simulink model "P702_NI_SoftECU"  (R2019a)
settings: Solver=ode1  StartTime=0.0  StopTime=Inf  FixedStep=0.001  RelTol=1e-3  EnableMultiTasking=on
PreLoadFcn:
  | run '.\VeriStand_BlockSet\NIVeriStandAddPaths.m'
undefined symbols (not defined in the file or in its folder): magnitude
libraries: simulink x83, simulink_extras x1
(part 61 of 76)

== system P702_NI_SoftECU/SoftECU/ABS/Logic/Wheel Direction ==
  note: 0: forward
      | 1: backward
      | 2: unknown
      | 3: fault
  note: 0: forward
      | 1: backward
      | 2: unknown
      | 3: fault
  WhlRl_W_Meas : Inport
  WhlRr_W_Meas : Inport  Port=2
  Backward : Constant
  Backward1 : Constant
  Forward : Constant  Value=0
  Forward1 : Constant  Value=0
  If Action Subsystem1 : Subsystem  TreatAsAtomicUnit=on
  If Action Subsystem2 : Subsystem  TreatAsAtomicUnit=on
  If Action Subsystem3 : Subsystem  TreatAsAtomicUnit=on
  If Action Subsystem4 : Subsystem  TreatAsAtomicUnit=on
  If Action Subsystem5 : Subsystem  TreatAsAtomicUnit=on
  If Action Subsystem6 : Subsystem  TreatAsAtomicUnit=on
  If_Rl : If  IfExpression=u1 == 0  ElseIfExpressions=u1 > 0, u1<0  ShowElse=off
  If_Rr : If  IfExpression=u1 == 0  ElseIfExpressions=u1 > 0, u1<0  ShowElse=off
  Merge : Merge  Inputs=3  InitialOutput=[0]
  Merge1 : Merge  Inputs=3  InitialOutput=[0]
  Unknown : Constant  Value=2
  Unknown1 : Constant  Value=2
  WhlDirRl_D_Actl : Outport
  WhlDirRr_D_Actl : Outport  Port=2
  wires:
  If_Rl/1 -> If Action Subsystem1/Action
  If Action Subsystem3/1(Out1) -> Merge/3
  If Action Subsystem2/1(Out1) -> Merge/2
  If Action Subsystem1/1(Out1) -> Merge/1
  If_Rl/3 -> If Action Subsystem3/Action
  If_Rl/2 -> If Action Subsystem2/Action
  Backward/1 -> If Action Subsystem3/1(In1)
  Forward/1 -> If Action Subsystem2/1(In1)
  Unknown/1 -> If Action Subsystem1/1(In1)
  If_Rr/1 -> If Action Subsystem4/Action
  If Action Subsystem6/1(Out1) -> Merge1/3
  If Action Subsystem5/1(Out1) -> Merge1/2
  If Action Subsystem4/1(Out1) -> Merge1/1
  If_Rr/3 -> If Action Subsystem6/Action
  If_Rr/2 -> If Action Subsystem5/Action
  Backward1/1 -> If Action Subsystem6/1(In1)
  Forward1/1 -> If Action Subsystem5/1(In1)
  Unknown1/1 -> If Action Subsystem4/1(In1)
  Merge/1 -> WhlDirRl_D_Actl/1
  Merge1/1 -> WhlDirRr_D_Actl/1
  WhlRl_W_Meas/1 -> If_Rl/1
  WhlRr_W_Meas/1 -> If_Rr/1

== system P702_NI_SoftECU/SoftECU/ABS/Logic/WheelSpeedCounterFL ==
  Omega : Inport
  8BitCounter : Constant  Value=255
  Abs : Abs
  Compare To Constant : simulink/Logic and Bit Operations/Compare To Constant  relop=>=  const=100*2*3.14  OutDataTypeStr=boolean  ZeroCross=off
  Divide : Product  Inputs=*/
  Integrator : Integrator  ExternalReset=rising
  Math Function1 : Math  Operator=mod  SaturateOnIntegerOverflow=on
  Memory : Memory
  RadperTick : Constant  Value=0.05
  Saturation1 : Saturate  UpperLimit=327.65  LowerLimit=0  OutDataTypeStr=double
  Counter : Outport
  wires:
  Integrator/1 -> Memory/1, Divide/1
  Abs/1 -> Saturation1/1
  RadperTick/1 -> Divide/2
  Divide/1 -> Math Function1/1
  8BitCounter/1 -> Math Function1/2
  Saturation1/1 -> Integrator/1
  Omega/1 -> Abs/1
  Math Function1/1 -> Counter/1
  Compare To Constant/1 -> Integrator/2
  Memory/1 -> Compare To Constant/1

== system P702_NI_SoftECU/SoftECU/ABS/Logic/WheelSpeedCounterFR ==
  Omega : Inport
  8BitCounter : Constant  Value=255
  Abs : Abs
  Compare To Constant : simulink/Logic and Bit Operations/Compare To Constant  relop=>=  const=100*2*3.14  OutDataTypeStr=boolean  ZeroCross=off
  Divide : Product  Inputs=*/
  Integrator : Integrator  ExternalReset=rising
  Math Function1 : Math  Operator=mod  SaturateOnIntegerOverflow=on
  Memory : Memory
  RadperTick : Constant  Value=0.05
  Saturation1 : Saturate  UpperLimit=327.65  LowerLimit=0  OutDataTypeStr=double
  Counter : Outport
  wires:
  Memory/1 -> Compare To Constant/1
  Compare To Constant/1 -> Integrator/2
  Math Function1/1 -> Counter/1
  Omega/1 -> Abs/1
  Saturation1/1 -> Integrator/1
  8BitCounter/1 -> Math Function1/2
  Divide/1 -> Math Function1/1
  RadperTick/1 -> Divide/2
  Abs/1 -> Saturation1/1
  Integrator/1 -> Divide/1, Memory/1

== system P702_NI_SoftECU/SoftECU/ABS/Logic/WheelSpeedCounterRL ==
  Omega : Inport
  8BitCounter : Constant  Value=255
  Abs : Abs
  Compare To Constant : simulink/Logic and Bit Operations/Compare To Constant  relop=>=  const=100*2*3.14  OutDataTypeStr=boolean  ZeroCross=off
  Divide : Product  Inputs=*/
  Integrator : Integrator  ExternalReset=rising
  Math Function1 : Math  Operator=mod  SaturateOnIntegerOverflow=on
  Memory : Memory
  RadperTick : Constant  Value=0.05
  Saturation1 : Saturate  UpperLimit=327.65  LowerLimit=0  OutDataTypeStr=double
  Counter : Outport
  wires:
  Memory/1 -> Compare To Constant/1
  Compare To Constant/1 -> Integrator/2
  Math Function1/1 -> Counter/1
  Omega/1 -> Abs/1
  Saturation1/1 -> Integrator/1
  8BitCounter/1 -> Math Function1/2
  Divide/1 -> Math Function1/1
  RadperTick/1 -> Divide/2
  Abs/1 -> Saturation1/1
  Integrator/1 -> Divide/1, Memory/1

== system P702_NI_SoftECU/SoftECU/ABS/Logic/WheelSpeedCounterRR ==
  Omega : Inport
  8BitCounter : Constant  Value=255
  Abs : Abs
  Compare To Constant : simulink/Logic and Bit Operations/Compare To Constant  relop=>=  const=100*2*3.14  OutDataTypeStr=boolean  ZeroCross=off
  Divide : Product  Inputs=*/
  Integrator : Integrator  ExternalReset=rising
  Math Function1 : Math  Operator=mod  SaturateOnIntegerOverflow=on
  Memory : Memory
  RadperTick : Constant  Value=0.05
  Saturation1 : Saturate  UpperLimit=327.65  LowerLimit=0  OutDataTypeStr=double
  Counter : Outport
  wires:
  Integrator/1 -> Memory/1, Divide/1
  Abs/1 -> Saturation1/1
  RadperTick/1 -> Divide/2
  Divide/1 -> Math Function1/1
  8BitCounter/1 -> Math Function1/2
  Saturation1/1 -> Integrator/1
  Omega/1 -> Abs/1
  Math Function1/1 -> Counter/1
  Compare To Constant/1 -> Integrator/2
  Memory/1 -> Compare To Constant/1

== system P702_NI_SoftECU/SoftECU/ABS/Logic/veh_chksum1 ==
  vspd : Inport
  qf : Inport  Port=2
  ctr : Inport  Port=3
  Bitwise Operator : simulink/Logic and Bit Operations/Bitwise Operator  logicop=AND  UseBitMask=on  BitMask=bin2dec('1111111100000000')  BitMaskRealWorld=Stored Integer
  Bitwise Operator1 : simulink/Logic and Bit Operations/Bitwise Operator  logicop=AND  UseBitMask=on  BitMask=bin2dec('0000000011111111')  BitMaskRealWorld=Stored Integer
  Bitwise Operator2 : simulink/Logic and Bit Operations/Bitwise Operator  logicop=XOR  UseBitMask=off  NumInputPorts=2  BitMask=bin2dec('11011001')  BitMaskRealWorld=Stored Integer
  Bitwise Operator4 : simulink/Logic and Bit Operations/Bitwise Operator  logicop=AND  UseBitMask=on  BitMask=uint32(255)  BitMaskRealWorld=Stored Integer
  Bitwise Operator5 : simulink/Logic and Bit Operations/Bitwise Operator  logicop=AND  UseBitMask=on  BitMask=uint32(255)  BitMaskRealWorld=Stored Integer
  Data Type Conversion : DataTypeConversion  OutDataTypeStr=uint16
  Data Type Conversion1 : DataTypeConversion  OutDataTypeStr=uint16
  Data Type Conversion{2,4,7,9..10} (5 alike) : DataTypeConversion  OutDataTypeStr=uint8
  Hil_flag : Constant
  Shift Arithmetic : ArithShift  BitShiftNumber=8
  Sum : Sum  Inputs=++++
  Switch : Switch  Criteria=u2 > Threshold
  constant1 : Constant  Value=255
  chksum : Outport
  wires:
  Data Type Conversion2/1 -> Bitwise Operator2/2
  constant1/1 -> Data Type Conversion2/1
  Sum/1 -> Bitwise Operator2/1
  Data Type Conversion4/1 -> Sum/1
  Data Type Conversion10/1 -> Sum/4
  Data Type Conversion9/1 -> Sum/3
  Data Type Conversion7/1 -> Sum/2
  ctr/1 -> Data Type Conversion10/1
  qf/1 -> Data Type Conversion9/1
  Bitwise Operator5/1 -> Data Type Conversion7/1
  Bitwise Operator4/1 -> Data Type Conversion4/1
  Shift Arithmetic/1 -> Bitwise Operator4/1
  Bitwise Operator/1 -> Shift Arithmetic/1
  Bitwise Operator1/1 -> Bitwise Operator5/1
  Switch/1 -> Bitwise Operator/1, Bitwise Operator1/1
  vspd/1 -> Data Type Conversion/1, Data Type Conversion1/1
  Hil_flag/1 -> Switch/2
  Data Type Conversion1/1 -> Switch/3
  Data Type Conversion/1 -> Switch/1
  Bitwise Operator2/1 -> chksum/1

== system P702_NI_SoftECU/SoftECU/ABS/Logic/veh_chksum2 ==
  vspd : Inport
  qf : Inport  Port=2
  ctr : Inport  Port=3
  Bitwise Operator : simulink/Logic and Bit Operations/Bitwise Operator  logicop=AND  UseBitMask=on  BitMask=bin2dec('1111111100000000')  BitMaskRealWorld=Stored Integer
  Bitwise Operator1 : simulink/Logic and Bit Operations/Bitwise Operator  logicop=AND  UseBitMask=on  BitMask=bin2dec('0000000011111111')  BitMaskRealWorld=Stored Integer
  Bitwise Operator2 : simulink/Logic and Bit Operations/Bitwise Operator  logicop=XOR  UseBitMask=off  NumInputPorts=2  BitMask=bin2dec('11011001')  BitMaskRealWorld=Stored Integer
  Bitwise Operator4 : simulink/Logic and Bit Operations/Bitwise Operator  logicop=AND  UseBitMask=on  BitMask=uint32(255)  BitMaskRealWorld=Stored Integer
  Bitwise Operator5 : simulink/Logic and Bit Operations/Bitwise Operator  logicop=AND  UseBitMask=on  BitMask=uint32(255)  BitMaskRealWorld=Stored Integer
  Data Type Conversion : DataTypeConversion  OutDataTypeStr=uint16
  Data Type Conversion1 : DataTypeConversion  OutDataTypeStr=uint16
  Data Type Conversion{2,4,7,9..10} (5 alike) : DataTypeConversion  OutDataTypeStr=uint8
  Hil_flag : Constant
  Shift Arithmetic : ArithShift  BitShiftNumber=8
  Sum : Sum  Inputs=++++
  Switch : Switch  Criteria=u2 > Threshold
  constant1 : Constant  Value=255
  chksum : Outport
  wires:
  Bitwise Operator2/1 -> chksum/1
  Data Type Conversion/1 -> Switch/1
  Data Type Conversion1/1 -> Switch/3
  Hil_flag/1 -> Switch/2
  vspd/1 -> Data Type Conversion1/1, Data Type Conversion/1
  Switch/1 -> Bitwise Operator1/1, Bitwise Operator/1
  Bitwise Operator1/1 -> Bitwise Operator5/1
  Bitwise Operator/1 -> Shift Arithmetic/1
  Shift Arithmetic/1 -> Bitwise Operator4/1
  Bitwise Operator4/1 -> Data Type Conversion4/1
  Bitwise Operator5/1 -> Data Type Conversion7/1
  qf/1 -> Data Type Conversion9/1
  ctr/1 -> Data Type Conversion10/1
  Data Type Conversion7/1 -> Sum/2
  Data Type Conversion9/1 -> Sum/3
  Data Type Conversion10/1 -> Sum/4
  Data Type Conversion4/1 -> Sum/1
  Sum/1 -> Bitwise Operator2/1
  constant1/1 -> Data Type Conversion2/1
  Data Type Conversion2/1 -> Bitwise Operator2/2

== system P702_NI_SoftECU/SoftECU/ABS/Mapping/ABS_BrkBst_Data ==
  In1 : Inport
  Bus Creator7 : BusCreator  Inputs=3
  Bus Selector3 : BusSelector  OutputSignals=BrkTot_Tq_RqDrv,BrkTotTqRqDrv_No_Cs,BrkTotTqRqDrv_No_Cnt
  Gain : Gain
  Gain1 : Gain
  Gain2 : Gain
  Out1 : Outport
  wires:
  Bus Selector3/2 -> Gain1/1  "<BrkTotTqRqDrv_No_Cs>"
  Bus Selector3/1 -> Gain/1  "<BrkTot_Tq_RqDrv>"
  In1/1 -> Bus Selector3/1
  Bus Creator7/1 -> Out1/1  "ABS_BrkBst_Data"
  Gain1/1 -> Bus Creator7/2  "BrkTotTqRqDrv_No_Cs"
  Gain/1 -> Bus Creator7/1  "BrkTot_Tq_RqDrv"
  Bus Selector3/3 -> Gain2/1  "<BrkTotTqRqDrv_No_Cnt>"
  Gain2/1 -> Bus Creator7/3  "BrkTotTqRqDrv_No_Cnt"

== system P702_NI_SoftECU/SoftECU/ABS/Mapping/Accel_Data ==
  In1 : Inport
  Bus Creator10 : BusCreator  Inputs=2
  Bus Selector3 : BusSelector  OutputSignals=VehLong2_A_Actl,VehLat2_A_Actl
  Gain : Gain
  Gain1 : Gain
  Out1 : Outport
  wires:
  Gain/1 -> Bus Creator10/1  "VehLong2_A_Actl"
  Gain1/1 -> Bus Creator10/2  "VehLat2_A_Actl"
  Bus Creator10/1 -> Out1/1  "Accel_Data"
  In1/1 -> Bus Selector3/1
  Bus Selector3/1 -> Gain/1  "<VehLong2_A_Actl>"
  Bus Selector3/2 -> Gain1/1  "<VehLat2_A_Actl>"

== system P702_NI_SoftECU/SoftECU/ABS/Mapping/BrakeSnData_3 ==
  In1 : Inport
  Bus Creator12 : BusCreator  Inputs=4
  Bus Selector3 : BusSelector  OutputSignals=VehYawComp_W_Actl,VehOverGnd_V_Est,VehLongComp_A_Actl,VehLatComp_A_Actl
  Gain{,1..3} (4 alike) : Gain
  Out1 : Outport
  wires:
  Gain1/1 -> Bus Creator12/2  "VehOverGnd_V_Est"
  Gain/1 -> Bus Creator12/1  "VehYawComp_W_Actl"
  Gain2/1 -> Bus Creator12/3  "VehLongComp_A_Actl"
  Gain3/1 -> Bus Creator12/4  "VehLatComp_A_Actl"
  Bus Creator12/1 -> Out1/1  "BrakeSnData_3"
  In1/1 -> Bus Selector3/1
  Bus Selector3/3 -> Gain2/1  "<VehLongComp_A_Actl>"
  Bus Selector3/2 -> Gain1/1  "<VehOverGnd_V_Est>"
  Bus Selector3/4 -> Gain3/1  "<VehLatComp_A_Actl>"
  Bus Selector3/1 -> Gain/1  "<VehYawComp_W_Actl>"

== system P702_NI_SoftECU/SoftECU/ABS/Mapping/BrakeSnData_4 ==
  In1 : Inport
  Bus Creator : BusCreator  Inputs=3
  Bus Selector3 : BusSelector  OutputSignals=VehVertComp_A_Actl,VehRolComp_W_Actl,BrkTot_Tq_RqDrv
  Gain : Gain
  Gain1 : Gain
  Gain2 : Gain
  Out1 : Outport
  wires:
  Gain/1 -> Bus Creator/1  "VehVertComp_A_Actl"
  Bus Creator/1 -> Out1/1  "BrakeSnData_4"
  Gain1/1 -> Bus Creator/2  "VehRolComp_W_Actl"
  Bus Selector3/1 -> Gain/1  "<VehVertComp_A_Actl>"
  Bus Selector3/2 -> Gain1/1  "<VehRolComp_W_Actl>"
  In1/1 -> Bus Selector3/1
  Bus Selector3/3 -> Gain2/1  "<BrkTot_Tq_RqDrv>"
  Gain2/1 -> Bus Creator/3  "BrkTot_Tq_Actl"

== system P702_NI_SoftECU/SoftECU/ABS/Mapping/BrakeSnData_5 ==
  In1 : Inport
  Bus Creator : BusCreator  Inputs=1
  Bus Selector3 : BusSelector  OutputSignals=SteWhlComp_An_Est
  Gain : Gain
  Out1 : Outport
  wires:
  In1/1 -> Bus Selector3/1
  Bus Selector3/1 -> Gain/1  "<SteWhlComp_An_Est>"
  Bus Creator/1 -> Out1/1  "BrakeSnData_5"
  Gain/1 -> Bus Creator/1  "SteWhlComp_An_Est"

== system P702_NI_SoftECU/SoftECU/ABS/Mapping/BrakeSysFeatures ==
  In1 : Inport
  Bus Creator5 : BusCreator  Inputs=3
  Bus Selector3 : BusSelector  OutputSignals=Veh_V_ActlBrk,VehVActlBrk_No_Cs,VehVActlBrk_No_Cnt
  Gain : Gain
  Gain1 : Gain
  Gain2 : Gain
  Out1 : Outport
  wires:
  Bus Creator5/1 -> Out1/1  "BrakeSysFeatures"
  Gain/1 -> Bus Creator5/1  "Veh_V_ActlBrk"
  In1/1 -> Bus Selector3/1
  Bus Selector3/1 -> Gain/1  "<Veh_V_ActlBrk>"
  Bus Selector3/2 -> Gain1/1  "<VehVActlBrk_No_Cs>"
  Bus Selector3/3 -> Gain2/1  "<VehVActlBrk_No_Cnt>"
  Gain1/1 -> Bus Creator5/2  "VehVActlBrk_No_Cs"
  Gain2/1 -> Bus Creator5/3  "VehVActlBrk_No_Cnt"

== system P702_NI_SoftECU/SoftECU/ABS/Mapping/BrakeSysFeatures_2 ==
  In1 : Inport
  Bus Creator7 : BusCreator  Inputs=3
  Bus Selector3 : BusSelector  OutputSignals=BpedMove_D_Actl,BpedMove_No_Cs,BpedMove_No_Cnt
  Gain : Gain
  Gain1 : Gain
  Gain2 : Gain
  Out1 : Outport
  wires:
  Gain2/1 -> Bus Creator7/3  "BpedMove_No_Cnt"
  Bus Selector3/3 -> Gain2/1  "<BpedMove_No_Cnt>"
  Gain/1 -> Bus Creator7/1  "BpedMove_D_Actl"
  Gain1/1 -> Bus Creator7/2  "BpedMove_No_Cs"
  Bus Creator7/1 -> Out1/1  "BrakeSysFeatures_2"
  In1/1 -> Bus Selector3/1
  Bus Selector3/1 -> Gain/1  "<BpedMove_D_Actl>"
  Bus Selector3/2 -> Gain1/1  "<BpedMove_No_Cs>"

== system P702_NI_SoftECU/SoftECU/ABS/Mapping/DesiredTorqBrk ==
  In1 : Inport
  Bus Creator11 : BusCreator  Inputs=10
  Bus Selector3 : BusSelector  OutputSignals=AccBrkPrchgActv_B_Actl,AccBrkActv_B_Actl,AccStopActv_B_ActlBrk,CmbbBrkPrchg_B_Actl,CmbbBaSensInc_B_Actl,CmbbBrkDecel_B_Actl,VehicleStationary,VehLongOvrGnd_A_Est,AccBrkTotTqMn_B_Actl
  Gain{,1..9} (10 alike) : Gain
  Out1 : Outport
  wires:
  Gain8/1 -> Bus Creator11/9  "VehLongOvrGnd_A_Est"
  Bus Creator11/1 -> Out1/1  "DesiredTorqBrk"
  Gain1/1 -> Bus Creator11/2  "AccBrkActv_B_Actl"
  Gain/1 -> Bus Creator11/1  "AccBrkPrchgActv_B_Actl"
  Gain2/1 -> Bus Creator11/3  "AccStopActv_B_ActlBrk"
  Gain3/1 -> Bus Creator11/4  "CmbbBrkPrchg_B_Actl"
  Gain4/1 -> Bus Creator11/5  "CmbbBaSensInc_B_Actl"
  Gain5/1 -> Bus Creator11/6  "CmbbBrkDecel_B_Actl"
  Gain6/1 -> Bus Creator11/7  "VehicleStationary"
  In1/1 -> Bus Selector3/1
  Bus Selector3/4 -> Gain3/1  "<CmbbBrkPrchg_B_Actl>"
  Bus Selector3/2 -> Gain1/1  "<AccBrkActv_B_Actl>"
  Bus Selector3/1 -> Gain/1  "<AccBrkPrchgActv_B_Actl>"
  Bus Selector3/3 -> Gain2/1  "<AccStopActv_B_ActlBrk>"
  Bus Selector3/5 -> Gain4/1  "<CmbbBaSensInc_B_Actl>"
  Bus Selector3/6 -> Gain5/1  "<CmbbBrkDecel_B_Actl>"
  Bus Selector3/7 -> Gain7/1, Gain6/1  "<VehicleStationary>"
  Bus Selector3/8 -> Gain8/1  "<VehLongOvrGnd_A_Est>"
  Bus Selector3/9 -> Gain9/1  "<AccBrkTotTqMn_B_Actl>"
  Gain9/1 -> Bus Creator11/10  "AccBrkTotTqMn_B_Actl"
  Gain7/1 -> Bus Creator11/8  "VehStop_D_Stat"

== system P702_NI_SoftECU/SoftECU/ABS/Mapping/ToCarSim ==
  In1 : Inport
  Bus Creator : BusCreator  Inputs=1
  Bus Selector3 : BusSelector  OutputSignals=ABSPhysical.MCPressure
  Out1 : Outport
  wires:
  In1/1 -> Bus Selector3/1
  Bus Creator/1 -> Out1/1  "ToCarSim"
  Bus Selector3/1 -> Bus Creator/1  "<MCPressure>"

== system P702_NI_SoftECU/SoftECU/ABS/Mapping/WheelData ==
  In1 : Inport
  Bus Creator7 : BusCreator  Inputs=2
  Bus Selector3 : BusSelector  OutputSignals=WhlDirRl_D_Actl,WhlDirRr_D_Actl
  Gain : Gain
  Gain1 : Gain
  Out1 : Outport
  wires:
  Gain/1 -> Bus Creator7/1  "WhlDirRl_D_Actl"
  Gain1/1 -> Bus Creator7/2  "WhlDirRr_D_Actl"
  Bus Creator7/1 -> Out1/1  "WheelData"
  In1/1 -> Bus Selector3/1
  Bus Selector3/1 -> Gain/1  "<WhlDirRl_D_Actl>"
  Bus Selector3/2 -> Gain1/1  "<WhlDirRr_D_Actl>"

== system P702_NI_SoftECU/SoftECU/ABS/Mapping/WheelSpeed ==
  In1 : Inport
  Bus Creator6 : BusCreator  Inputs=8
  Bus Selector3 : BusSelector  OutputSignals=WhlFl_W_Meas,WhlFr_W_Meas,WhlRl_W_Meas,WhlRr_W_Meas,WhlRotatFl_No_Cnt,WhlRotatFr_No_Cnt,WhlRotatRl_No_Cnt,WhlRotatRr_No_Cnt
  Gain{,1..7} (8 alike) : Gain
  Out1 : Outport
  wires:
  In1/1 -> Bus Selector3/1
  Gain/1 -> Bus Creator6/1  "WhlFl_W_Meas"
  Gain1/1 -> Bus Creator6/2  "WhlFr_W_Meas"
  Gain2/1 -> Bus Creator6/3  "WhlRl_W_Meas"
  Gain3/1 -> Bus Creator6/4  "WhlRr_W_Meas"
  Bus Creator6/1 -> Out1/1  "WheelSpeed"
  Bus Selector3/2 -> Gain1/1  "<WhlFr_W_Meas>"
  Bus Selector3/1 -> Gain/1  "<WhlFl_W_Meas>"
  Bus Selector3/3 -> Gain2/1  "<WhlRl_W_Meas>"
  Bus Selector3/4 -> Gain3/1  "<WhlRr_W_Meas>"
  Bus Selector3/8 -> Gain7/1  "<WhlRotatRr_No_Cnt>"
  Bus Selector3/7 -> Gain6/1  "<WhlRotatRl_No_Cnt>"
  Bus Selector3/5 -> Gain4/1  "<WhlRotatFl_No_Cnt>"
  Bus Selector3/6 -> Gain5/1  "<WhlRotatFr_No_Cnt>"
  Gain7/1 -> Bus Creator6/8  "WhlRotatRr_No_Cnt"
  Gain6/1 -> Bus Creator6/7  "WhlRotatRl_No_Cnt"
  Gain4/1 -> Bus Creator6/5  "WhlRotatFl_No_Cnt"
  Gain5/1 -> Bus Creator6/6  "WhlRotatFr_No_Cnt"

== system P702_NI_SoftECU/SoftECU/ABS/Mapping/Yaw_Data ==
  In1 : Inport
  Bus Creator9 : BusCreator  Inputs=1
  Bus Selector3 : BusSelector  OutputSignals=VehYaw_W_Actl
  Gain : Gain
  Out1 : Outport
  wires:
  Gain/1 -> Bus Creator9/1  "VehYaw_W_Actl"
  Bus Creator9/1 -> Out1/1  "Yaw_Data"
  In1/1 -> Bus Selector3/1
  Bus Selector3/1 -> Gain/1  "<VehYaw_W_Actl>"

== system P702_NI_SoftECU/SoftECU/BCM/Logic/GGCC_Config_Mgmt_ID ==
  note: VIN:
      | 17 characters as ASCII vector
      |
      | AxleRatio:
      | Min = 0.01
      | Max = 655.34
      | Res = 0.01
      |
      | TireCircumference:
      | Min = 1
      | Max = 65534
      | Res = 1
      | Unit = mm
      |
      | RCMAuxId:
      | 2 bytes
      |
      | LowSpeedCmbbCfg:
      | 1 = Without Low Speed CMbB
      | 2 = Low Speed CMbB
      |
      | FuelCfg:
      | 1 = Gasoline
      | 2 = Diesel
      | 3 = Gas/Electric Hybrid
      | 4 = Hydrogen Fuel Cell
      | 5 = Diesel/Electric Hybrid
      | 6 = Compressed Natural Gas
      | 7 = Electric Only
      |
      | AccCfg:
      | 1 = Without Cruise Control
      | 2 = Cruise Control
      | 3 = Adaptive Cruise Control
      | 4 = Adaptive Cruise Control Stop & Go
      |
      | DriveCfg:
      | 1 = Without 4WD
      | 2 = Selectable 4WD
      | 3 = Permanent 4WD
      | 4 = AWD
      |
      | DriveSideCfg:
      | 1 = Left Hand Drive
      | 2 = Right Hand Drive
      |
      | GearboxCfg:
      | 1 = Manual
      | 2 = Automatic
  note: KunalP: VINCalculation Modified by BrianTamm
  AccCfg : Constant  Value=4
  AxleRatio : Constant  Value=3.21
  Bus Creator : BusCreator  Inputs=8
  Bus Creator1 : BusCreator  Inputs=1
  CmbbCfg : Constant  Value=3
  DriveCfg : Constant
  DriveSideCfg : Constant
  FuelCfg : Constant
  GearboxCfg : Constant  Value=2
  LowSpeedCmbbCfg : Constant
  MUX_delay : UnitDelay  SampleTime=0.2  HasFrameUpgradeWarning=on
  RCMAuxId : Constant  Value=hex2dec('20C3')
  Rate Transition1 : RateTransition
  Terminator{,1..5} (6 alike) : Terminator
  TireCircumference : Constant  Value=2534
  VIN : Constant  Value=double('ABCDEFGHIJKLMNOPQ')  VectorParams1D=off  OutDataTypeStr=double
  VIN_Calculation : MATLAB Function  TreatAsAtomicUnit=on
  Out1 : Outport
  wires:
  Bus Creator1/1 -> Out1/1  "GGCC_Config_Mgmt_ID"
  MUX_delay/1 -> VIN_Calculation/12(MUX_in)
  VIN_Calculation/9(MUX_out) -> Rate Transition1/1
  VIN_Calculation/2(Byte_1) -> Bus Creator/2
  VIN_Calculation/3(Byte_2) -> Bus Creator/3
  VIN_Calculation/4(Byte_3) -> Bus Creator/4
  VIN_Calculation/5(Byte_4) -> Bus Creator/5
  VIN_Calculation/6(Byte_5) -> Bus Creator/6
  VIN_Calculation/7(Byte_6) -> Bus Creator/7
  VIN_Calculation/8(Byte_7) -> Bus Creator/8
  Rate Transition1/1 -> MUX_delay/1
  Bus Creator/1 -> Bus Creator1/1  "VehicleGGCCData"
  VIN_Calculation/1(Byte_0) -> Bus Creator/1
  VIN/1 -> VIN_Calculation/1(VIN)
  AxleRatio/1 -> VIN_Calculation/2(AxleRatio)
  TireCircumference/1 -> VIN_Calculation/3(TireCircumference)
  RCMAuxId/1 -> VIN_Calculation/4(RCMAuxId)
  LowSpeedCmbbCfg/1 -> VIN_Calculation/5(LowSpeedCmbbCfg)
  FuelCfg/1 -> VIN_Calculation/6(FuelCfg)
  AccCfg/1 -> VIN_Calculation/7(AccCfg)
  CmbbCfg/1 -> VIN_Calculation/8(CmbbCfg)
  DriveCfg/1 -> VIN_Calculation/9(DriveCfg)
  DriveSideCfg/1 -> VIN_Calculation/10(DriveSideCfg)
  GearboxCfg/1 -> VIN_Calculation/11(GearboxCfg)
  VIN_Calculation/10(C000_out) -> Terminator/1
  VIN_Calculation/11(C100_out) -> Terminator1/1
  VIN_Calculation/12(C101_out) -> Terminator2/1
  VIN_Calculation/13(C102_out) -> Terminator3/1
  VIN_Calculation/14(C104_out) -> Terminator4/1
  VIN_Calculation/15(C110_out) -> Terminator5/1

== system P702_NI_SoftECU/SoftECU/BCM/Logic/IgnitionState ==
  In : Inport
  Accessory : Constant  Value=2
  Bus Creator : BusCreator  Inputs=1
  Constant : Constant  Value=2
  If : If  IfExpression=u1 <= 0  ElseIfExpressions=u1 == 1, u1 == 2, u1 == 3
  If Action Subsystem1 : Subsystem  TreatAsAtomicUnit=on
  If Action Subsystem2 : Subsystem  TreatAsAtomicUnit=on
  If Action Subsystem3 : Subsystem  TreatAsAtomicUnit=on
  If Action Subsystem4 : Subsystem  TreatAsAtomicUnit=on
  If Action Subsystem5 : Subsystem  TreatAsAtomicUnit=on
  Invalid : Constant  Value=15
  Merge : Merge  Inputs=5  InitialOutput=[0]
  Off : Constant
  Run : Constant  Value=4
  Start : Constant  Value=8
  Terminator : Terminator
  Out : Outport
  wires:
  Merge/1 -> Bus Creator/1  "IgnitionStatus"
  Off/1 -> If Action Subsystem1/1(In1)
  Accessory/1 -> If Action Subsystem2/1(In1)
  Run/1 -> If Action Subsystem3/1(In1)
  Start/1 -> If Action Subsystem4/1(In1)
  Invalid/1 -> If Action Subsystem5/1(In1)
  If/2 -> If Action Subsystem2/Action
  If/5 -> If Action Subsystem5/Action
  If/3 -> If Action Subsystem3/Action
  If/4 -> If Action Subsystem4/Action
  If Action Subsystem1/1(Out1) -> Merge/1
  If Action Subsystem2/1(Out1) -> Merge/2
  If Action Subsystem3/1(Out1) -> Merge/3
  If Action Subsystem4/1(Out1) -> Merge/4
  If Action Subsystem5/1(Out1) -> Merge/5
  If/1 -> If Action Subsystem1/Action
  In/1 -> Terminator/1
  Constant/1 -> If/1
  Bus Creator/1 -> Out/1  "Ignition"

== system P702_NI_SoftECU/SoftECU/BCM/Logic/OdometerValues ==
  In : Inport
  Bus Creator : BusCreator  Inputs=2
  Bus Selector2 : BusSelector  OutputSignals=s_Vehicle[m]
  Constant : Constant  Value=1000
  Constant2 : Constant  Value=1000
  Derivative : Derivative
  Divide : Product  Inputs=*/
  If : If  IfExpression=u1 <= 0
  If Action Subsystem1 : Subsystem  TreatAsAtomicUnit=on
  If Action Subsystem4 : Subsystem  TreatAsAtomicUnit=on
  Merge : Merge  InitialOutput=[0]
  Off : Constant  Value=0
  Start : Constant
  Start1 : Constant  Value=0.5
  Sum : Sum  Inputs=++|
  Variable Time Delay : VariableTransportDelay  MaximumDelay=10  MaximumPoints=10240
  Out : Outport
  wires:
  In/1 -> Bus Selector2/1
  Bus Creator/1 -> Out/1  "OdometerValues"
  Bus Selector2/1 -> Divide/1  "<s_Vehicle[m]>"
  Constant/1 -> Divide/2
  Divide/1 -> Sum/2
  Sum/1 -> Bus Creator/1, Derivative/1  "OdometerMasterValue"
  Merge/1 -> Variable Time Delay/1
  Off/1 -> If Action Subsystem1/1(In1)
  Start/1 -> If Action Subsystem4/1(In1)
  If/2 -> If Action Subsystem4/Action
  If Action Subsystem1/1(Out1) -> Merge/1
  If Action Subsystem4/1(Out1) -> Merge/2
  If/1 -> If Action Subsystem1/Action
  Derivative/1 -> If/1
  Start1/1 -> Variable Time Delay/2
  Variable Time Delay/1 -> Bus Creator/2  "OdometerMasterValue_UB"
  Constant2/1 -> Sum/1

== system P702_NI_SoftECU/SoftECU/BCM/Mapping/BodyEngGateway_2 ==
  In1 : Inport
  Ground : Ground
  Terminator : Terminator
  Out1 : Outport
  wires:
  In1/1 -> Terminator/1
  Ground/1 -> Out1/1

== system P702_NI_SoftECU/SoftECU/BCM/Mapping/BodyInfo_3 ==
  In : Inport
  Bus Creator : BusCreator  Inputs=1
  Bus Selector : BusSelector  OutputSignals=Ignition.IgnitionStatus
  Gain : Gain
  Out : Outport
  wires:
  Gain/1 -> Bus Creator/1  "Ignition_Status"
  Bus Creator/1 -> Out/1  "BodyInfo_3"
  In/1 -> Bus Selector/1
  Bus Selector/1 -> Gain/1  "<IgnitionStatus>"

== system P702_NI_SoftECU/SoftECU/BCM/Mapping/Cluster_Info1 ==
  In : Inport
  Bus Creator : BusCreator  Inputs=2
  Bus Selector2 : BusSelector  OutputSignals=OdometerValues.OdometerMasterValue,OdometerValues.OdometerMasterValue_UB
  Gain : Gain
  Gain1 : Gain
  Out : Outport
  wires:
  Gain1/1 -> Bus Creator/2  "OdometerMasterValue_UB"
  Gain/1 -> Bus Creator/1  "OdometerMasterValue"
  Bus Selector2/2 -> Gain1/1  "<OdometerMasterValue_UB>"
  Bus Selector2/1 -> Gain/1  "<OdometerMasterValue>"
  Bus Creator/1 -> Out/1  "Cluster_Info1"
  In/1 -> Bus Selector2/1

== system P702_NI_SoftECU/SoftECU/BCM/Mapping/GGCC_Config_Mgmt_ID ==
  In1 : Inport
  Bus Creator : BusCreator  Inputs=8
  Bus Selector : BusSelector  OutputSignals=GGCC_Config_Mgmt_ID.VehicleGGCCData.Byte_0,GGCC_Config_Mgmt_ID.VehicleGGCCData.Byte_1,GGCC_Config_Mgmt_ID.VehicleGGCCData.Byte_2,GGCC_Config_Mgmt_ID.VehicleGGCCData.Byte_3,GGCC_Config_Mgmt_ID.VehicleGGCCData.Byte_4,GGCC_Config_Mgmt_ID.VehicleGGCCData.Byte_5,GGCC_Config_Mgmt_ID.VehicleGGCCData.Byte_6,GGCC_Config_Mgmt_ID.VehicleGGCCData.Byte_7
  Out1 : Outport
  wires:
  In1/1 -> Bus Selector/1
  Bus Creator/1 -> Out1/1  "GGCC_Config_Mgmt_ID"
  Bus Selector/3 -> Bus Creator/3  "<Byte_2>"
  Bus Selector/6 -> Bus Creator/6  "<Byte_5>"
  Bus Selector/4 -> Bus Creator/4  "<Byte_3>"
  Bus Selector/2 -> Bus Creator/2  "<Byte_1>"
  Bus Selector/8 -> Bus Creator/8  "<Byte_7>"
  Bus Selector/7 -> Bus Creator/7  "<Byte_6>"
  Bus Selector/5 -> Bus Creator/5  "<Byte_4>"
  Bus Selector/1 -> Bus Creator/1  "<Byte_0>"

== system P702_NI_SoftECU/SoftECU/BCM/Mapping/Gear_Shift_By_Wire ==
  In1 : Inport
  Ground : Ground
  Terminator : Terminator
  Out1 : Outport
  wires:
  In1/1 -> Terminator/1
  Ground/1 -> Out1/1

== system P702_NI_SoftECU/SoftECU/BCM/Mapping/KeyStates ==
  In : Inport
  Ground : Ground
  Terminator : Terminator
  Out : Outport
  wires:
  In/1 -> Terminator/1
  Ground/1 -> Out/1

== system P702_NI_SoftECU/SoftECU/BCM/Mapping/Personality_BCM2_Data ==
  note: Han: the update rate of Personality_BCM2_Data is 1 Hz
  Bus Creator : BusCreator  Inputs=1
  Counter Limited : simulink/Sources/Counter Limited  uplimit=255  tsamp=1
  Data Type Conversion : DataTypeConversion  OutDataTypeStr=uint8
  Out : Outport
  wires:
  Bus Creator/1 -> Out/1  "Personality_BCM2_Data"
  Counter Limited/1 -> Data Type Conversion/1
  Data Type Conversion/1 -> Bus Creator/1  "RecallEvent_No_Cnt"

== system P702_NI_SoftECU/SoftECU/DSMC/Logic/Compute_DrvEngageLevel_No_Cs ==
  DrvEngLvlConfid_D_Stat : Inport
  DrvEngageLevel_D_Stat : Inport  Port=2
  DrvEngageLevel_No_Cnt : Inport  Port=3
  Bitwise Operator1 : simulink/Logic and Bit Operations/Bitwise Operator  logicop=AND  UseBitMask=on  BitMask=bin2dec('0000000011111111')  BitMaskRealWorld=Stored Integer
  Bitwise Operator2 : simulink/Logic and Bit Operations/Bitwise Operator  logicop=NOT  UseBitMask=off  BitMask=bin2dec('11011001')  BitMaskRealWorld=Stored Integer
  Bitwise Operator4 : simulink/Logic and Bit Operations/Bitwise Operator  logicop=AND  UseBitMask=on  BitMask=bin2dec('0000000011111111')  BitMaskRealWorld=Stored Integer
  Data Type Conversion{1,3..6} (5 alike) : DataTypeConversion  OutDataTypeStr=uint8
  DrvEngageLevel_No_Cnt_In : simulink/Sources/Counter Limited  uplimit=15  tsamp=-1
  Sig_DrvEngageLevel_No_Cnt_CheckinLogic : S-Function  Priority=1  FunctionName=NIVeriStandIO  Parameters=width dtype portnum stime stype btype  SFunctionDeploymentMode=off  EnableBusSupport=off  mask(NI VeriStand Outport){portnum=1, width=-1, stime=-1, dtype=auto, stype=auto, btype=0}
      mask prompts: portnum "Port number:"; width "Port dimensions (-1 for dynamically sized):"; stime "Sample time (-1 for inherited):"; dtype "Data type:"; stype "Signal type:"; btype "Block type:"
      mask help: Use this outport on any level of nested subsystems to allow NI VeriStand software to map signals to it.
      mask init:
      | NIVeriStandIO_init;
      settings: CopyFcn=NIVeriStand_MDL_functions('', 'IO_copy');  DeleteFcn=NIVeriStand_MDL_functions('', 'IO_delete');  MoveFcn=set_param(gcb, 'Mask', 'on');
      mask Callback portnum: NIVeriStand_MDL_functions('', 'IO_setportnum');
      mask TypeOptions dtype: auto | double | single | int8 | uint8 | int16 | uint16 | int32 | uint32 | boolean
      mask Callback dtype: NIVeriStand_MDL_functions('', 'IO_booleansignal');
      mask TypeOptions stype: auto | real | complex
      mask Display:
      | patch([-x x], [-y y], [.90980 .81960 .32156]);
      | plot([xrad -x x xrad], [yrad -y y yrad]);
      | fprintf('NI Out%d', portnum);
  Sum : Sum  Inputs=+++
  Terminator : Terminator
  DrvEngageLevel_No_Cs : Outport
  DrvEngageLevel_No_Cnt1 : Outport  Port=2
  wires:
  DrvEngLvlConfid_D_Stat/1 -> Data Type Conversion6/1
  Bitwise Operator1/1 -> Data Type Conversion3/1
  DrvEngageLevel_D_Stat/1 -> Data Type Conversion1/1
  Sum/1 -> Bitwise Operator2/1
  Bitwise Operator2/1 -> DrvEngageLevel_No_Cs/1  "DrvEngageLevel_No_Cs"
  Data Type Conversion3/1 -> Sum/2  "DrvEngageLevel_D_Stat"
  Data Type Conversion4/1 -> Sum/3, Sig_DrvEngageLevel_No_Cnt_CheckinLogic/1, DrvEngageLevel_No_Cnt1/1  "DrvEngageLevel_No_Cnt"
  Data Type Conversion5/1 -> Sum/1  "DrvEngLvlConfid_D_Stat"
  Bitwise Operator4/1 -> Data Type Conversion5/1
  Data Type Conversion6/1 -> Bitwise Operator4/1
  Data Type Conversion1/1 -> Bitwise Operator1/1
  DrvEngageLevel_No_Cnt/1 -> Terminator/1
  DrvEngageLevel_No_Cnt_In/1 -> Data Type Conversion4/1  "DrvEngageevel_No_Cnt"

== system P702_NI_SoftECU/SoftECU/DSMC/Mapping/DrvStatMonData ==
  In1 : Inport
  Bus Creator : BusCreator  Inputs=3
  Bus Selector : BusSelector  OutputSignals=DrvEngLvlConfid_D_Stat,DrvEngageLevel_No_Cs,DrvEngageLevel_No_Cnt
  Gain : Gain
  Gain1 : Gain
  Gain2 : Gain
  Out1 : Outport
  wires:
  In1/1 -> Bus Selector/1
  Gain/1 -> Bus Creator/2  "DrvEngageLevel_No_Cs"
  Gain1/1 -> Bus Creator/3  "DrvEngageLevel_No_Cnt"
  Bus Selector/2 -> Gain/1  "<DrvEngageLevel_No_Cs>"
  Bus Selector/3 -> Gain1/1  "<DrvEngageLevel_No_Cnt>"
  Gain2/1 -> Bus Creator/1  "DrvEngLvlConfid_D_Stat"
  Bus Selector/1 -> Gain2/1  "<DrvEngLvlConfid_D_Stat>"
  Bus Creator/1 -> Out1/1  "DrvStatMonData"

== system P702_NI_SoftECU/SoftECU/ECM/Mapping/EngBrakeData ==
  In1 : Inport
  In2 : Inport  Port=2
  AccDeny_B : S-Function  Priority=2  FunctionName=NIVeriStandIO  Parameters=width dtype portnum stime stype btype  SFunctionDeploymentMode=off  EnableBusSupport=off  mask(NI VeriStand Inport){portnum=2, width=-1, stime=-1, dtype=auto, stype=auto, btype=1}
      mask prompts: portnum "Port number:"; width "Port dimensions (-1 for dynamically sized):"; stime "Sample time (-1 for inherited):"; dtype "Data type:"; stype "Signal type:"; btype "Block type:"
      mask help: Use this inport on any level of nested subsystems to allow NI VeriStand software to map signals to it.
      mask init:
      | NIVeriStandIO_init;
      settings: CopyFcn=NIVeriStand_MDL_functions('', 'IO_copy');  DeleteFcn=NIVeriStand_MDL_functions('', 'IO_delete');  MoveFcn=set_param(gcb, 'Mask', 'on');
      mask Callback portnum: NIVeriStand_MDL_functions('', 'IO_setportnum');
      mask TypeOptions dtype: auto | double | single | int8 | uint8 | int16 | uint16 | int32 | uint32 | boolean
      mask Callback dtype: NIVeriStand_MDL_functions('', 'IO_booleansignal');
      mask TypeOptions stype: auto | real | complex
      mask Display:
      | patch([-x x], [-y y], [.90980 .81960 .32156]);
      | plot([xrad -x x xrad], [yrad -y y yrad]);
      | fprintf('NI In%d', portnum);
  Acc_veh_reset : S-Function  Priority=1  FunctionName=NIVeriStandIO  Parameters=width dtype portnum stime stype btype  SFunctionDeploymentMode=off  EnableBusSupport=off  mask(NI VeriStand Inport){portnum=1, width=-1, stime=-1, dtype=auto, stype=auto, btype=1}
      mask prompts: portnum "Port number:"; width "Port dimensions (-1 for dynamically sized):"; stime "Sample time (-1 for inherited):"; dtype "Data type:"; stype "Signal type:"; btype "Block type:"
      mask help: Use this inport on any level of nested subsystems to allow NI VeriStand software to map signals to it.
      mask init:
      | NIVeriStandIO_init;
      settings: CopyFcn=NIVeriStand_MDL_functions('', 'IO_copy');  DeleteFcn=NIVeriStand_MDL_functions('', 'IO_delete');  MoveFcn=set_param(gcb, 'Mask', 'on');
      mask Callback portnum: NIVeriStand_MDL_functions('', 'IO_setportnum');
      mask TypeOptions dtype: auto | double | single | int8 | uint8 | int16 | uint16 | int32 | uint32 | boolean
      mask Callback dtype: NIVeriStand_MDL_functions('', 'IO_booleansignal');
      mask TypeOptions stype: auto | real | complex
      mask Display:
      | patch([-x x], [-y y], [.90980 .81960 .32156]);
      | plot([xrad -x x xrad], [yrad -y y yrad]);
      | fprintf('NI In%d', portnum);
  Bus Creator : BusCreator  Inputs=4
  Bus Selector1 : BusSelector  OutputSignals=ADAS.ACCDATA.CmbbEngTqMn_B_Rq,ADAS.ACCDATA.AccCancl_B_Rq,RealPCM.user_channel.PCM_status_user_input,RealPCM.EngBrakeData.CcStat_D_Actl,ADAS.ACCDATA.AccPrpl_A_Rq,ADAS.ACCDATA.AccStopStat_B_Rq,ADAS.ACCDATA.AccBrkPrchg_B_Rq
  Bus Selector3 : BusSelector  OutputSignals=V_x_veh_COG[km/h]
  ReValueStates : Subsystem
      mask Display: disp('RevalueStates')
  Out1 : Outport
  tag scope: A=global
  wires:
  Bus Creator/1 -> Out1/1
  Bus Selector1/1 -> Bus Creator/1  "<CmbbEngTqMn_B_Rq>"
  In1/1 -> Bus Selector1/1
  Bus Selector1/2 -> ReValueStates/1(ACCCancl_B_Rq)  "<AccCancl_B_Rq>"
  Bus Selector1/6 -> ReValueStates/7(AccStopStat_B_Rq)  "<AccStopStat_B_Rq>"
  Bus Selector1/4 -> ReValueStates/3(CcStat_D_Actl)  "<CcStat_D_Actl>"
  Bus Selector1/5 -> ReValueStates/4(ACC_Prpl_A_Req)  "<AccPrpl_A_Rq>"
  ReValueStates/1(AccStopMde_D_Rq) -> Bus Creator/2  "ACCStopMde_D_Rq"
  ReValueStates/3(Cc_Stat_D_Actl) -> Bus Creator/4, [A]  "Cc_Stat_D_Actl"
  Bus Selector1/3 -> ReValueStates/2(PCM_status_user_input)  "<PCM_status_user_input>"
  Acc_veh_reset/1 -> ReValueStates/5(ACC_veh_reset)
  In2/1 -> Bus Selector3/1
  Bus Selector3/1 -> ReValueStates/6(VehSpeed)  "<V_x_veh_COG[km/h]>"
  Bus Selector1/7 -> ReValueStates/8(AccBrkPrChg_B_Rq)  "<AccBrkPrchg_B_Rq>"
  ReValueStates/2(PrplTqMnSat_B_Actl) -> Bus Creator/3  "PrplTqMnSat_B_Actl"
  AccDeny_B/1 -> ReValueStates/9(AccDeny_B)

== system P702_NI_SoftECU/SoftECU/ECM/Mapping/EngVehicleSpThrottle ==
  note: Duplicated from PCM -not mapped to CAN
  In1 : Inport
  Bus Creator : BusCreator  Inputs=1
  Bus Selector2 : BusSelector  OutputSignals=Engine_RPM[rpm]
  Gain : Gain
  Out1 : Outport
  wires:
  In1/1 -> Bus Selector2/1
  Bus Creator/1 -> Out1/1
  Bus Selector2/1 -> Gain/1  "<Engine_RPM[rpm]>"
  Gain/1 -> Bus Creator/1  "EngAout_N_Actl"

== system P702_NI_SoftECU/SoftECU/ECM/Mapping/EngVehicleSpThrottle2 ==
  note: Duplicated from PCM -not mapped to CAN
  In2 : Inport
  Bus Creator : BusCreator  Inputs=1
  Bus Selector : BusSelector  OutputSignals=V_x_veh_COG[km/h]
  Gain : Gain
  Out1 : Outport
  wires:
  Bus Creator/1 -> Out1/1
  Gain/1 -> Bus Creator/1  "Veh_V_ActlEng"
  Bus Selector/1 -> Gain/1  "<V_x_veh_COG[km/h]>"
  In2/1 -> Bus Selector/1

== system P702_NI_SoftECU/SoftECU/MRR/Logic/Array2Bus ==
  MappedData : Inport
  NumOfDetections : Inport  Port=2
  Add : Sum  Inputs=+++
  BusCreator1 : BusCreator  Inputs=5
  BusCreator2 : BusCreator  Inputs=5
  BusCreator3 : BusCreator  Inputs=5
  BusCreatorMessages : BusCreator  Inputs=3
  BusCreatorMessages1 : BusCreator  Inputs=2
  Demux1 : Demux  Outputs=5
  Demux2 : Demux  Outputs=5
  Demux3 : Demux  Outputs=5
  Saturation : Saturate  UpperLimit=1  LowerLimit=0
  Selector1 : Selector  NumberOfDimensions=2  IndexOptions=Index vector (dialog),Index vector (dialog)  Indices=1,[1:5]  OutputSizes=3,1
  Selector2 : Selector  NumberOfDimensions=2  IndexOptions=Index vector (dialog),Index vector (dialog)  Indices=2,[1:5]  OutputSizes=3,1
  Selector3 : Selector  NumberOfDimensions=2  IndexOptions=Index vector (dialog),Index vector (dialog)  Indices=3,[1:5]  OutputSizes=3,1
  Terminator : Terminator
  MRR_Data : Outport
  wires:
  MappedData/1 -> Selector1/1, Selector3/1, Selector2/1
  Selector1/1 -> Demux1/1
  Demux1/1 -> BusCreator1/1  "CAN_DET_RANGE_01"
  Demux1/2 -> BusCreator1/2  "CAN_DET_RANGE_RATE_01"
  Demux1/3 -> BusCreator1/3  "CAN_DET_AZIMUTH_01"
  Demux1/4 -> BusCreator1/4, Add/3  "CAN_DET_VALID_LEVEL_01"
  Demux1/5 -> BusCreator1/5  "CAN_DET_AMPLITUDE_01"
  Selector2/1 -> Demux2/1
  Demux2/1 -> BusCreator2/1  "CAN_DET_RANGE_02"
  Demux2/2 -> BusCreator2/2  "CAN_DET_RANGE_RATE_02"
  Demux2/3 -> BusCreator2/3  "CAN_DET_AZIMUTH_02"
  Demux2/4 -> BusCreator2/4, Add/2  "CAN_DET_VALID_LEVEL_02"
  Demux2/5 -> BusCreator2/5  "CAN_DET_AMPLITUDE_02"
  Selector3/1 -> Demux3/1
  Demux3/1 -> BusCreator3/1  "CAN_DET_RANGE_03"
  Demux3/2 -> BusCreator3/2  "CAN_DET_RANGE_RATE_03"
  Demux3/3 -> BusCreator3/3  "CAN_DET_AZIMUTH_03"
  Demux3/4 -> BusCreator3/4, Add/1  "CAN_DET_VALID_LEVEL_03"
  Demux3/5 -> BusCreator3/5  "CAN_DET_AMPLITUDE_03"
  BusCreator1/1 -> BusCreatorMessages/1  "MRR_Detection_001"
  BusCreator2/1 -> BusCreatorMessages/2  "MRR_Detection_002"
  BusCreator3/1 -> BusCreatorMessages/3  "MRR_Detection_003"
  BusCreatorMessages/1 -> BusCreatorMessages1/1  "MRR_Detection"
  BusCreatorMessages1/1 -> MRR_Data/1
  NumOfDetections/1 -> Terminator/1  "NumOfDetections"
  Add/1 -> [NumOfDetections]
  Saturation/1 -> BusCreatorMessages1/2  "NumOfDetections"
  [NumOfDetections] -> Saturation/1

== system P702_NI_SoftECU/SoftECU/MRR/Logic/Bus2Array ==
  RadarSensor : Inport
  Azimuth : Subsystem
  Range : Subsystem
  Range_Rate : Subsystem
  Dist_Fellows : Outport
  v_Rel_Fellows : Outport  Port=2
  Angle_Hor_Rel_Fellows : Outport  Port=3
  wires:
  RadarSensor/1 -> Range/1(In1), Range_Rate/1(In1), Azimuth/1(In1)
  Range/1(Out1) -> Dist_Fellows/1
  Range_Rate/1(Out1) -> v_Rel_Fellows/1
  Azimuth/1(Out1) -> Angle_Hor_Rel_Fellows/1

== system P702_NI_SoftECU/SoftECU/PCM/Logic1/Compute ApedPosPcActl CheckSum ==
  note: Take from Carsim PCM pedalpercentage: now connected to Throttle Percentage
  ApedPos_Pc_ActlArb : Inport
  Add : Sum  Inputs=++++
  "ApedPosPcActl_D_Qf " : Constant  Value=3
  Bitwise Operator : simulink/Logic and Bit Operations/Bitwise Operator  logicop=AND  UseBitMask=on  BitMask=bin2dec('1111111100000000')  BitMaskRealWorld=Stored Integer
  Bitwise Operator1 : simulink/Logic and Bit Operations/Bitwise Operator  logicop=AND  UseBitMask=on  BitMask=bin2dec('0000000011111111')  BitMaskRealWorld=Stored Integer
  Bitwise Operator2 : simulink/Logic and Bit Operations/Bitwise Operator  logicop=NOT  UseBitMask=off  BitMask=bin2dec('11110000')  BitMaskRealWorld=Stored Integer
  Bus Selector : BusSelector  OutputSignals=Throttle[percentage]
  Counter Limited : simulink/Sources/Counter Limited  uplimit=15  tsamp=-1
  Data Type Conversion : DataTypeConversion  OutDataTypeStr=uint8
  Data Type Conversion1 : DataTypeConversion  OutDataTypeStr=uint8
  Data Type Conversion2 : DataTypeConversion  OutDataTypeStr=uint16
  Data Type Conversion3 : DataTypeConversion  OutDataTypeStr=uint16
  Data Type Conversion4 : DataTypeConversion  OutDataTypeStr=uint8
  Factor : Constant  Value=0.1
  Gain : Gain
  Gain1 : Gain
  Product : Product  Inputs=*/
  Shift Arithmetic : ArithShift  BitShiftNumber=8
  ApedPosPcActl_No_Cs : Outport
  ApedPos_Pc_ActlArb_No_Cnt : Outport  Port=2
  ApedPos_Pc_Actl_D_Qf : Outport  Port=3
  wires:
  Bitwise Operator2/1 -> ApedPosPcActl_No_Cs/1  "ApedPosPcActl_No_Cs"
  Counter Limited/1 -> Data Type Conversion/1
  Data Type Conversion/1 -> Add/4, Gain/1  "ApedPosPcActl_No_Cnt"
  ApedPos_Pc_ActlArb/1 -> Bus Selector/1
  "ApedPosPcActl_D_Qf "/1 -> Data Type Conversion1/1, Gain1/1  "ApedPos_Pc_Actl_D_Qf"
  Gain/1 -> ApedPos_Pc_ActlArb_No_Cnt/1  "ApedPosPcActl_No_Cnt"
  Gain1/1 -> ApedPos_Pc_Actl_D_Qf/1  "ApedPos_Pc_Actl_D_Qf"
  Add/1 -> Data Type Conversion4/1
  Bitwise Operator/1 -> Shift Arithmetic/1
  Bitwise Operator1/1 -> Add/2
  Data Type Conversion1/1 -> Add/3
  Data Type Conversion2/1 -> Bitwise Operator/1
  Data Type Conversion3/1 -> Bitwise Operator1/1
  Data Type Conversion4/1 -> Bitwise Operator2/1
  Shift Arithmetic/1 -> Add/1
  Product/1 -> Data Type Conversion2/1, Data Type Conversion3/1
  Bus Selector/1 -> Product/1  "<Throttle[percentage]>"
  Factor/1 -> Product/2

== system P702_NI_SoftECU/SoftECU/PCM/Logic1/Compute GearPos_No CheckSum ==
  GearLvr_D_Actl : Inport
  CAN : Inport  Port=2
  Add : Sum  Inputs=++++++
  Bitwise Operator2 : simulink/Logic and Bit Operations/Bitwise Operator  logicop=NOT  UseBitMask=off  BitMask=bin2dec('11110000')  BitMaskRealWorld=Stored Integer
  Bus Selector : BusSelector  OutputSignals=ECM_DIESEL PCM PCM_HEV.PowertrainData_10.GearPos_D_Actl,ECM_DIESEL PCM PCM_HEV.PowertrainData_10.GearPos_D_Trg,ECM_DIESEL PCM PCM_HEV.PowertrainData_10.TrnPrkSys_D_Actl,ECM_DIESEL PCM PCM_HEV.PowertrainData_10.TrnRng_D_Rq
  Counter Limited : simulink/Sources/Counter Limited  uplimit=15  tsamp=-1
  Data Type Conversion{,1..8} (9 alike) : DataTypeConversion  OutDataTypeStr=uint8
  GearPos_D_Actl : Constant  Value=15
  GearPos_D_Trg : Constant  Value=15
  Terminator{,1..3} (4 alike) : Terminator
  TrnPrkSys_D_Actl : Constant  Value=0
  TrnRng_D_Rq : Constant  Value=14
  GearPos_No_Cs : Outport
  GearPos_No_Cnt : Outport  Port=2
  GearLvr_D_ActlDrv : Outport  Port=3
  wires:
  Data Type Conversion4/1 -> Bitwise Operator2/1
  Data Type Conversion1/1 -> GearPos_No_Cnt/1  "GearPos_No_Cnt"
  Bitwise Operator2/1 -> GearPos_No_Cs/1  "GearPos_No_Cs"
  Add/1 -> Data Type Conversion4/1
  GearLvr_D_Actl/1 -> Data Type Conversion2/1, Data Type Conversion3/1
  Counter Limited/1 -> Data Type Conversion/1
  Data Type Conversion/1 -> Add/6, Data Type Conversion1/1
  Data Type Conversion2/1 -> GearLvr_D_ActlDrv/1  "GearLvr_D_ActlDrv"
  Data Type Conversion3/1 -> Add/1
  Data Type Conversion5/1 -> Add/2
  Data Type Conversion6/1 -> Add/3
  Data Type Conversion7/1 -> Add/4
  Data Type Conversion8/1 -> Add/5
  CAN/1 -> Bus Selector/1
  GearPos_D_Actl/1 -> Terminator/1
  GearPos_D_Trg/1 -> Terminator1/1
  TrnPrkSys_D_Actl/1 -> Terminator2/1
  TrnRng_D_Rq/1 -> Terminator3/1
  Bus Selector/2 -> Data Type Conversion6/1  "<GearPos_D_Trg>"
  Bus Selector/3 -> Data Type Conversion7/1  "<TrnPrkSys_D_Actl>"
  Bus Selector/1 -> Data Type Conversion5/1  "<GearPos_D_Actl>"
  Bus Selector/4 -> Data Type Conversion8/1  "<TrnRng_D_Rq>"

== system P702_NI_SoftECU/SoftECU/PCM/Logic1/Compute PrplWhlTotTqRq CheckSum ==
  PrplWhlTot_Tq_Rq : Inport
  Add : Sum  Inputs=+++
  Bitwise Operator : simulink/Logic and Bit Operations/Bitwise Operator  logicop=AND  UseBitMask=on  BitMask=bin2dec('1111111100000000')  BitMaskRealWorld=Stored Integer
  Bitwise Operator1 : simulink/Logic and Bit Operations/Bitwise Operator  logicop=AND  UseBitMask=on  BitMask=bin2dec('0000000011111111')  BitMaskRealWorld=Stored Integer
  Bitwise Operator2 : simulink/Logic and Bit Operations/Bitwise Operator  logicop=NOT  UseBitMask=off  BitMask=bin2dec('11110000')  BitMaskRealWorld=Stored Integer
  Counter Limited : simulink/Sources/Counter Limited  uplimit=15  tsamp=-1
  Data Type Conversion : DataTypeConversion  OutDataTypeStr=uint8
  Data Type Conversion1 : DataTypeConversion  OutDataTypeStr=uint8
  Data Type Conversion2 : DataTypeConversion  OutDataTypeStr=uint16
  Data Type Conversion3 : DataTypeConversion  OutDataTypeStr=uint16
  Data Type Conversion4 : DataTypeConversion  OutDataTypeStr=uint8
  Factor : Constant  Value=4
  Offset : Constant  Value=131072
  Product : Product  Inputs=*/
  Shift Arithmetic : ArithShift  BitShiftNumber=8
  Sum : Sum  Inputs=|++
  PrplWhlTotTqRq_No_Cs : Outport
  PrplWhlTot_Tq_Rq_No_Cnt : Outport  Port=2
  wires:
  Data Type Conversion/1 -> Add/3, Data Type Conversion1/1
  Counter Limited/1 -> Data Type Conversion/1
  Product/1 -> Data Type Conversion2/1, Data Type Conversion3/1
  Add/1 -> Data Type Conversion4/1
  Bitwise Operator2/1 -> PrplWhlTotTqRq_No_Cs/1  "PrplWhlTotTqRq_No_Cs"
  Data Type Conversion1/1 -> PrplWhlTot_Tq_Rq_No_Cnt/1  "PrplWhlTot_Tq_Rq_No_Cnt"
  Bitwise Operator/1 -> Shift Arithmetic/1
  Bitwise Operator1/1 -> Add/2
  Data Type Conversion2/1 -> Bitwise Operator/1
  Data Type Conversion3/1 -> Bitwise Operator1/1
  Data Type Conversion4/1 -> Bitwise Operator2/1
  Shift Arithmetic/1 -> Add/1
  PrplWhlTot_Tq_Rq/1 -> Sum/1
  Offset/1 -> Sum/2
  Sum/1 -> Product/1
  Factor/1 -> Product/2

== system P702_NI_SoftECU/SoftECU/PCM/Logic1/EngVehSpeed ==
  VehSp : Inport
  Bus Creator : BusCreator  Inputs=3
  Bus Selector : BusSelector  OutputSignals=V_total_Vehicle[km/h]
  Bus Selector7 : BusSelector  OutputSignals=Gear[]
  CalcGearRvrseActv : Subsystem
  Gain : Gain
  Vset_CruiseControl : S-Function  Priority=1  FunctionName=NIVeriStandIO  Parameters=width dtype portnum stime stype btype  SFunctionDeploymentMode=off  EnableBusSupport=off  mask(NI VeriStand Inport){portnum=1, width=-1, stime=-1, dtype=auto, stype=auto, btype=1}
      mask prompts: portnum "Port number:"; width "Port dimensions (-1 for dynamically sized):"; stime "Sample time (-1 for inherited):"; dtype "Data type:"; stype "Signal type:"; btype "Block type:"
      mask help: Use this inport on any level of nested subsystems to allow NI VeriStand software to map signals to it.
      mask init:
      | NIVeriStandIO_init;
      settings: CopyFcn=NIVeriStand_MDL_functions('', 'IO_copy');  DeleteFcn=NIVeriStand_MDL_functions('', 'IO_delete');  MoveFcn=set_param(gcb, 'Mask', 'on');
      mask Callback portnum: NIVeriStand_MDL_functions('', 'IO_setportnum');
      mask TypeOptions dtype: auto | double | single | int8 | uint8 | int16 | uint16 | int32 | uint32 | boolean
      mask Callback dtype: NIVeriStand_MDL_functions('', 'IO_booleansignal');
      mask TypeOptions stype: auto | real | complex
      mask Display:
      | patch([-x x], [-y y], [.90980 .81960 .32156]);
      | plot([xrad -x x xrad], [yrad -y y yrad]);
      | fprintf('NI In%d', portnum);
  SpeedInformation : Outport
  wires:
  Vset_CruiseControl/1 -> Bus Creator/3  "Veh_V_RqCcSet"
  CalcGearRvrseActv/1(Out1) -> Bus Creator/2  "CalcGearRvrseActv"
  Bus Selector7/1 -> CalcGearRvrseActv/1(In1)  "<Gear[]>"
  VehSp/1 -> Bus Selector/1, Bus Selector7/1  "EngineSpeed"
  Bus Selector/1 -> Gain/1  "<V_total_Vehicle[km/h]>"
  Bus Creator/1 -> SpeedInformation/1  "EngVehSpeed"
  Gain/1 -> Bus Creator/1  "VehicleSpeed_No"
